simulink model "tvc_rocket"  (R2023a)
settings: Solver=VariableStepAuto  StartTime=0.0  StopTime=10.0  RelTol=1e-3
settings Model: Creator=Vinesh  LastModifiedBy=Vinesh

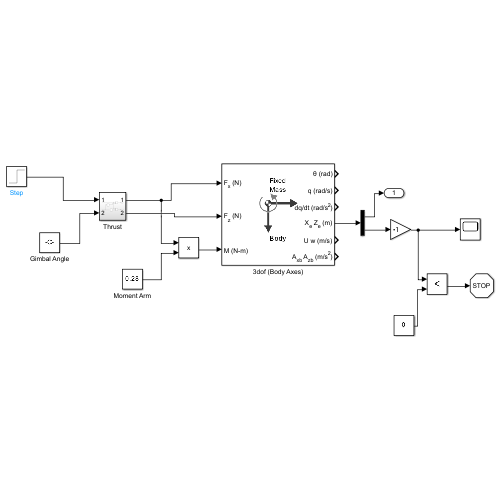
[thumbnail: Simulink's stored preview of the top-level diagram]
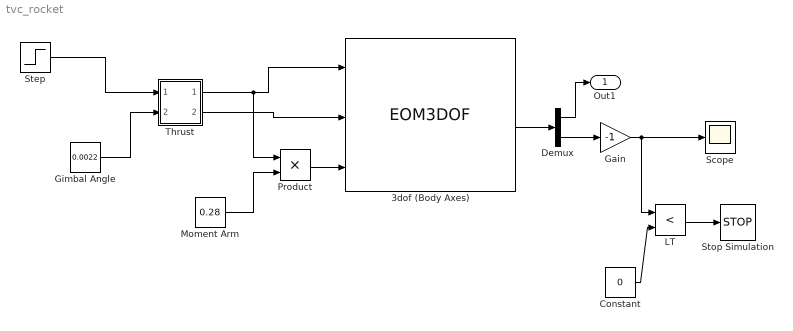
== system tvc_rocket ==
  3dof (Body Axes) : EOM3DOF  v_ini=0  mass=0.543  Iyy=0.048
  Constant : Constant  Value=0
  Demux : Demux  Outputs=2
  Gain : Gain  Gain=-1
  Gimbal Angle : Constant  Value=0.0022  OutDataTypeStr=Inherit: Inherit via back propagation
  LT : RelationalOperator  Operator=<  OutDataTypeStr=boolean  RndMeth=Simplest  InputSameDT=off
  Moment Arm : Constant  Value=0.28  OutDataTypeStr=Inherit: Inherit via back propagation
  Product : Product
  Scope : Scope
  Step : Step  Time=2  Before=-15  After=0  SampleTime=0
  Stop Simulation : Stop
  Thrust : Subsystem
  Out1 : Outport
  wires:
  Gain/1 -> Scope/1, LT/1
  3dof (Body Axes)/4 -> Demux/1
  Demux/2 -> Gain/1
  Constant/1 -> LT/2
  LT/1 -> Stop Simulation/1
  Demux/1 -> Out1/1
  Thrust/1(Out3) -> Product/1, 3dof (Body Axes)/1
  Thrust/2(Out2) -> 3dof (Body Axes)/2
  Product/1 -> 3dof (Body Axes)/3
  Moment Arm/1 -> Product/2
  Gimbal Angle/1 -> Thrust/2(In2)
  Step/1 -> Thrust/1(In1)

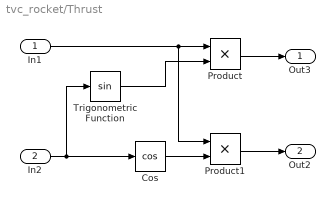
== system tvc_rocket/Thrust ==
  In1 : Inport
  In2 : Inport  Port=2
  Cos : Trigonometry  Operator=cos
  Product : Product
  Product1 : Product
  Trigonometric Function : Trigonometry
  Out3 : Outport
  Out2 : Outport  Port=2
  wires:
  In1/1 -> Product1/1, Product/1
  Cos/1 -> Product1/2
  In2/1 -> Cos/1, Trigonometric Function/1
  Trigonometric Function/1 -> Product/2
  Product1/1 -> Out2/1
  Product/1 -> Out3/1
